simulink model "SIR_simulink"  (R2023b)
settings: Solver=VariableStepAuto  StartTime=0.0  StopTime=1000  RelTol=1e-3
values from neighbouring files (symbols this model uses):
  b = 0.004    [ese3a.m]
  delta = 0.1    [ese3a.m]
  g = 0.04    [ese3a.m]
  mu = 1e-3    (= 0.001)    [ese3a.m]
settings Model: Creator=stefa  LastModifiedBy=stefa

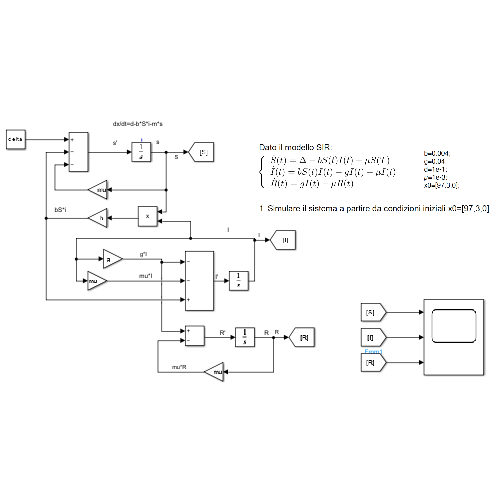
[thumbnail: Simulink's stored preview of the top-level diagram]
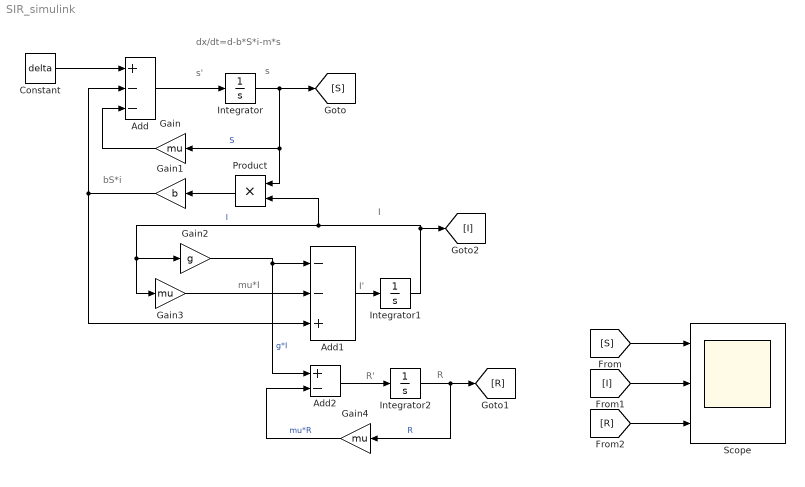
== system SIR_simulink ==
  note: mu*I
  note: R
  note: R'
  note: I'
  note: I
  note: bS*i
  note: s'
  note: s
  note: dx/dt=d-b*S*i-m*s
  Add : Sum  Inputs=+--
  Add1 : Sum  Inputs=--+
  Add2 : Sum  Inputs=+-
  Constant : Constant  Value=delta
  Gain : Gain  Gain=mu
  Gain1 : Gain  Gain=b
  Gain2 : Gain  Gain=g
  Gain3 : Gain  Gain=mu
  Gain4 : Gain  Gain=mu
  Integrator : Integrator  InitialCondition=97
  Integrator1 : Integrator  InitialCondition=3
  Integrator2 : Integrator
  Product : Product
  Scope : Scope  NumInputPorts=3
  wires:
  Constant/1 -> Add/1
  Gain/1 -> Add/3
  Integrator/1 -> Product/1, Gain/1, [S]  "S"
  Add/1 -> Integrator/1
  Product/1 -> Gain1/1
  Gain3/1 -> Add1/2
  Gain2/1 -> Add2/1, Add1/1  "g*I"
  Gain1/1 -> Add1/3, Add/2
  Add1/1 -> Integrator1/1
  Integrator1/1 -> Product/2, Gain3/1, Gain2/1, [I]  "I"
  Gain4/1 -> Add2/2  "mu*R"
  Add2/1 -> Integrator2/1
  Integrator2/1 -> [R], Gain4/1  "R"
  [S] -> Scope/1
  [I] -> Scope/2
  [R] -> Scope/3
